simulink model "Integrated_model"  (R2017b)
settings: Solver=VariableStepAuto  StartTime=0.0  StopTime=10.0  RelTol=1e-3
model workspace (MAT data in the model file):
  H_Speed = 3600
  H_limit = 2500
  L_limit = 0
  inputVoltage = 5
  nBitConverter = 10
undefined symbols (not defined in the file): sigbuilder_block
libraries: simulink x2
(part 1 of 2)
settings Model: Creator=ECoDe_user11  LastModifiedBy=ECoDe_user11
settings DebuggingCC: SignalInfNanChecking=warning  ParameterUnderflowMsg=warning  UniqueDataStoreMsg=warning  StrictBusMsg=ErrorOnBusTreatedAsVector

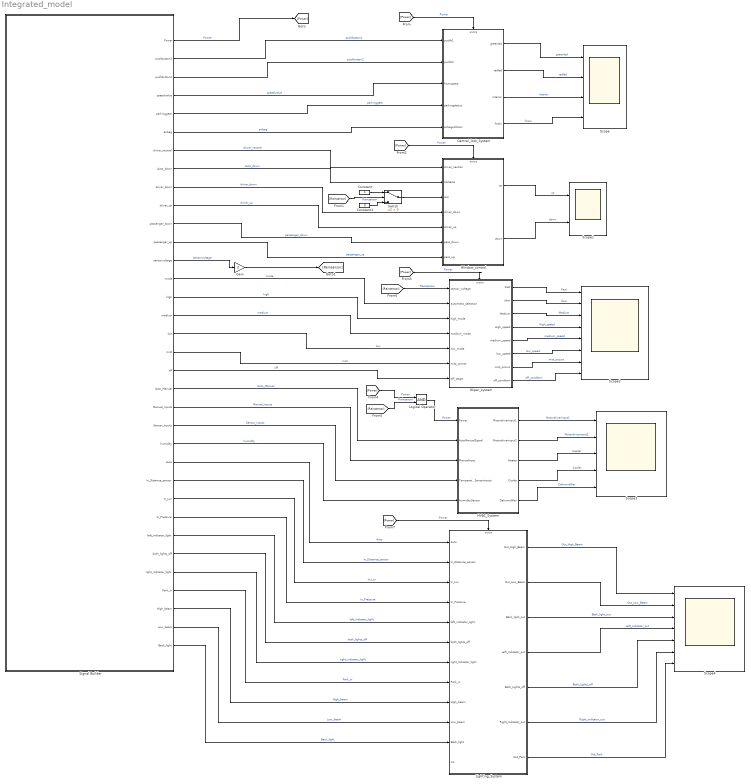
== system Integrated_model ==
  Central_lock_System : Subsystem
  Constant : Constant
  Constant1 : Constant  Value=0
  Gain : Gain  Gain=2
  HVAC_System : Subsystem
  Lighting_System : Subsystem
  Logical Operator : Logic  AllPortsSameDT=off  OutDataTypeStr=boolean
  Scope : Scope  NumInputPorts=4
  Scope1 : Scope  NumInputPorts=2
  Scope2 : Scope  NumInputPorts=8
  Scope3 : Scope  NumInputPorts=5
  Scope4 : Scope  NumInputPorts=7
  Signal Builder : Subsystem  Tag=STV Subsys  LoadFcn=sigbuilder_block('load');  StartFcn=sigbuilder_block('start');  StopFcn=sigbuilder_block('stop');  ClipboardFcn=sigbuilder_block('clipboard');  mask(Sigbuilder block){tuvar=[0:10]}
      mask help: Simulink:masks:SigbuilderBlock_MD
      mask init:
      | if ~strcmp(get_param(bdroot(gcbh),'SimulationStatus'),'stopped') tuvar = sigbuilder_block('maskInit'); end
      settings: CopyFcn=sigbuilder_block('copy');  DeleteFcn=sigbuilder_block('delete');  ModelCloseFcn=sigbuilder_block('modelClose');  PreSaveFcn=sigbuilder_block('preSave');  PauseFcn=sigbuilder_block('pause');  ContinueFcn=sigbuilder_block('continue');  NameChangeFcn=sigbuilder_block('namechange');  OpenFcn=sigbuilder_block('open',[437.25 159 550.5 363.75 ]);  CloseFcn=sigbuilder_block('close');
      mask Display: plot(0, 0, 100, 100,[2, 2, 32, 32, 2], [68, 8, 8, 68, 68],[32, 2], [38, 38], [32, 19, 2],[53, 60, 44], [32, 17, 17, 2],[16, 16, 31, 31]);txt = getActiveGroup(gcbh);text(2, 100, txt,'verticalAlignment', 'top');
  Switch : Switch  Criteria=u2 > Threshold
  Window_control : Subsystem
  Wiper_system : Subsystem
  wires:
  Signal Builder/2(pushbutton1) -> Central_lock_System/1(pushb1)  "pushbutton1"
  Signal Builder/3(pushbutton2) -> Central_lock_System/2(pushb2)  "pushbutton2"
  Signal Builder/4(speedvalue) -> Central_lock_System/3(fromspeed)  "speedvalue"
  Signal Builder/5(parkinggear) -> Central_lock_System/4(parkingstatus)  "parkinggear"
  Signal Builder/6(airbag) -> Central_lock_System/5(airbagcollision)  "airbag"
  Signal Builder/7(driver_neutral) -> Window_control/1(driver_neutral)  "driver_neutral"
  Signal Builder/8(Auto_down) -> Window_control/2(obstacle)  "Auto_down"
  Signal Builder/9(driver_down) -> Window_control/4(driver_down)  "driver_down"
  Signal Builder/10(driver_up) -> Window_control/5(driver_up)  "driver_up"
  Signal Builder/11(passenger_down) -> Window_control/6(pass_down)  "passenger_down"
  Signal Builder/12(passenger_up) -> Window_control/7(pass_up)  "passenger_up"
  Signal Builder/1(Power) -> [Power]  "Power"
  Signal Builder/13(sensorvoltage) -> Gain/1  "sensorvoltage"
  [Power] -> Central_lock_System/Enable  "Power"
  [Power] -> Window_control/Enable  "Power"
  [Power] -> Wiper_system/Enable  "Power"
  [Power] -> Logical Operator/1  "Power"
  [Rainsensor] -> Logical Operator/2  "Rainsensor"
  Switch/1 -> Window_control/3(rain)
  [Rainsensor] -> Switch/2  "Rainsensor"
  Constant/1 -> Switch/1
  Constant1/1 -> Switch/3
  Gain/1 -> [Rainsensor]
  Logical Operator/1 -> HVAC_System/1(Power)  "Power"
  [Rainsensor] -> Wiper_system/1(sensor_voltage)  "Rainsensor"
  Signal Builder/14(mode) -> Wiper_system/2(automatic_selection)  "mode"
  Signal Builder/15(high) -> Wiper_system/3(high_mode)  "high"
  Signal Builder/16(medium) -> Wiper_system/4(medium_mode)  "medium"
  Signal Builder/17(low) -> Wiper_system/5(low_mode)  "low"
  Signal Builder/18(mist) -> Wiper_system/6(mist_comes)  "mist"
  Signal Builder/19(off) -> Wiper_system/7(off_stage)  "off"
  Signal Builder/20(Auto_Manual) -> HVAC_System/2(AutoManualSignal)  "Auto_Manual"
  Signal Builder/21(Manual_inputs) -> HVAC_System/3(ManualInpts)  "Manual_inputs"
  Signal Builder/22(Sensor_inputs) -> HVAC_System/4(TemperatureSensorinputs)  "Sensor_inputs"
  Signal Builder/23(humidity) -> HVAC_System/5(HumiditySensor)  "humidity"
  [Power] -> Lighting_System/Enable  "Power"
  Signal Builder/24(Auto) -> Lighting_System/1(Auto)  "Auto"
  Signal Builder/25(In_Distance_sensor) -> Lighting_System/2(In_Distance_sensor)  "In_Distance_sensor"
  Signal Builder/26(In_Lux) -> Lighting_System/3(In_Lux)  "In_Lux"
  Signal Builder/27(In_Pressure) -> Lighting_System/4(In_Pressure)  "In_Pressure"
  Signal Builder/28(left_indicator_light) -> Lighting_System/5(left_indicator_light)  "left_indicator_light"
  Signal Builder/29(both_lights_off) -> Lighting_System/6(both_lights_off)  "both_lights_off"
  Signal Builder/30(right_indicator_light) -> Lighting_System/7(right_indicator_light)  "right_indicator_light"
  Signal Builder/31(Park_in) -> Lighting_System/8(Park_in)  "Park_in"
  Signal Builder/32(High_beam) -> Lighting_System/9(High_beam)  "High_beam"
  Signal Builder/33(Low_beam) -> Lighting_System/10(Low_beam)  "Low_beam"
  Signal Builder/34(Back_light) -> Lighting_System/11(Back_light)  "Back_light"
  Central_lock_System/1(greenled) -> Scope/1  "greenled"
  Central_lock_System/2(redled) -> Scope/2  "redled"
  Central_lock_System/3(interior) -> Scope/3  "interior"
  Central_lock_System/4(finalv) -> Scope/4  "finalv"
  Window_control/1(up) -> Scope1/1  "up"
  Window_control/2(down) -> Scope1/2  "down"
  Wiper_system/1(Fast) -> Scope2/1  "Fast"
  Wiper_system/2(slow) -> Scope2/2  "slow"
  Wiper_system/3(Medium) -> Scope2/3  "Medium"
  Wiper_system/4(High_speed) -> Scope2/4  "High_speed"
  Wiper_system/5(medium_speed) -> Scope2/5  "medium_speed"
  Wiper_system/6(low_speed) -> Scope2/6  "low_speed"
  Wiper_system/7(mist_occurs) -> Scope2/7  "mist_occurs"
  Wiper_system/8(off_condition) -> Scope2/8  "off_condition"
  HVAC_System/1(Motordriverinput1) -> Scope3/1  "Motordriverinput1"
  HVAC_System/2(Motordriverinput2) -> Scope3/2  "Motordriverinput2"
  HVAC_System/3(Heater) -> Scope3/3  "Heater"
  HVAC_System/4(Cooler) -> Scope3/4  "Cooler"
  HVAC_System/5(Dehumidifier) -> Scope3/5  "Dehumidifier"
  Lighting_System/1(Out_High_Beam) -> Scope4/1  "Out_High_Beam"
  Lighting_System/2(Out_Low_Beam) -> Scope4/2  "Out_Low_Beam"
  Lighting_System/3(Back_light_out) -> Scope4/3  "Back_light_out"
  Lighting_System/4(Left_indicator_out) -> Scope4/4  "Left_indicator_out"
  Lighting_System/5(Both_Lights_off) -> Scope4/5  "Both_Lights_off"
  Lighting_System/6(Right_indicator_out) -> Scope4/6  "Right_indicator_out"
  Lighting_System/7(Out_Park) -> Scope4/7  "Out_Park"

== system Integrated_model/Central_lock_System ==
  note: %REQUIRMENTS:
      | CENTRAL LOCKING SYSTEM
      | CONSISTS OF FOUR SUB SYSTEMS
      | SUB SYSTEM FOR LIGHTING
      | SUB SYSTEM FOR MANUAL
      | SUB SYSTEM FOR AUTOMATIC
      | SUB SYSTEM FOR EMERGENCY
      | INPUTS:
      | PUSHBUTTON1
      | PUSHBUTTON2
      | INPUTBASEDONSPEED
      | INPUTBASEDONPARKINGGEAR
      | AIRBAGINPUT
      | OUTPUTS:
      | LEDS AND INTERIORLIGHTS
      | LOCK AND UNLOCK STATUS
  pushb1 : Inport
  pushb2 : Inport  Port=2
  fromspeed : Inport  Port=3
  parkingstatus : Inport  Port=4
  airbagcollision : Inport  Port=5
  power : EnablePort
  main_locking_system : Subsystem
  greenled : Outport
  redled : Outport  Port=2
  interior : Outport  Port=3
  finalv : Outport  Port=4
  wires:
  fromspeed/1 -> main_locking_system/3(fromspeed)  "fromspeed"
  main_locking_system/2(redled) -> redled/1  "redled"
  main_locking_system/3(interior) -> interior/1  "interior"
  main_locking_system/4(finalv) -> finalv/1  "finalv"
  airbagcollision/1 -> main_locking_system/5(airbagcollision)  "airbagcollision"
  parkingstatus/1 -> main_locking_system/4(parkingstatus)  "parkingstatus"
  main_locking_system/1(greenled) -> greenled/1  "greenled"
  pushb2/1 -> main_locking_system/2(pushb2)  "pushb2"
  pushb1/1 -> main_locking_system/1(pushb1)  "pushb1"

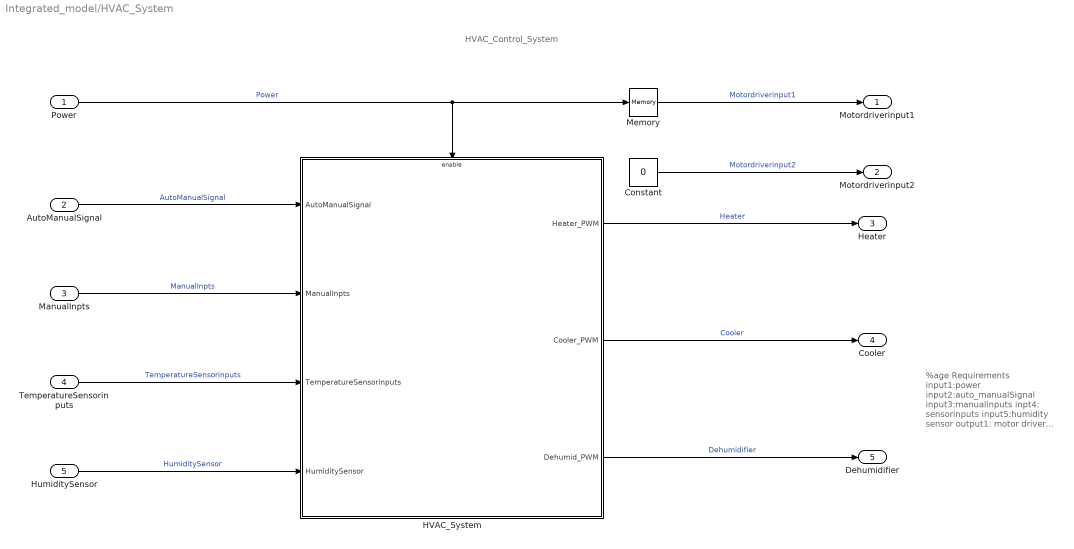
== system Integrated_model/HVAC_System ==
  note: HVAC_Control_System
  note: %age Requirements
      |
      | input1:power
      | input2:auto_manualSignal
      | input3:manualinputs
      | inpt4: sensorinputs
      | input5:humidity sensor
      | output1: motor driver output
      | output2: mptor driver output
      | output3: PWM for Heater
      | output4: PWM for Cooler
      | output5: PWM for Dehumidifier
  Power : Inport
  AutoManualSignal : Inport  Port=2
  ManualInpts : Inport  Port=3
  TemperatureSensorinputs : Inport  Port=4
  HumiditySensor : Inport  Port=5
  Constant : Constant  Value=0
  HVAC_System : Subsystem
  Memory : Memory
  Motordriverinput1 : Outport
  Motordriverinput2 : Outport  Port=2
  Heater : Outport  Port=3
  Cooler : Outport  Port=4
  Dehumidifier : Outport  Port=5
  wires:
  AutoManualSignal/1 -> HVAC_System/1(AutoManualSignal)  "AutoManualSignal"
  ManualInpts/1 -> HVAC_System/2(ManualInpts)  "ManualInpts"
  TemperatureSensorinputs/1 -> HVAC_System/3(TemperatureSensorinputs)  "TemperatureSensorinputs"
  Power/1 -> Memory/1, HVAC_System/Enable  "Power"
  HVAC_System/1(Heater_PWM) -> Heater/1  "Heater"
  HVAC_System/3(Dehumid_PWM) -> Dehumidifier/1  "Dehumidifier"
  HumiditySensor/1 -> HVAC_System/4(HumiditySensor)  "HumiditySensor"
  HVAC_System/2(Cooler_PWM) -> Cooler/1  "Cooler"
  Constant/1 -> Motordriverinput2/1  "Motordriverinput2"
  Memory/1 -> Motordriverinput1/1  "Motordriverinput1"

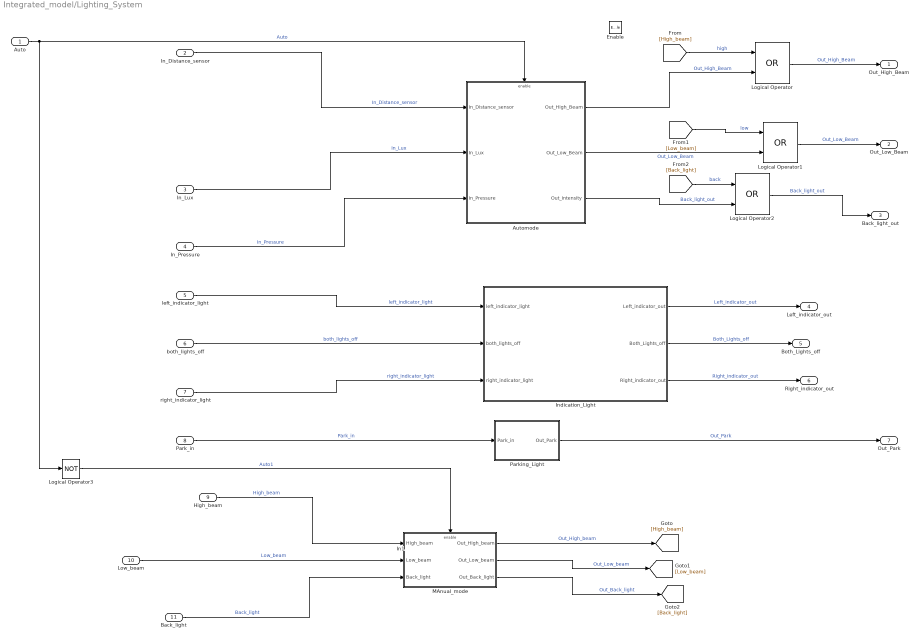
== system Integrated_model/Lighting_System ==
  Auto : Inport
  In_Distance_sensor : Inport  Port=2
  In_Lux : Inport  Port=3
  In_Pressure : Inport  Port=4
  left_indicator_light : Inport  Port=5
  both_lights_off : Inport  Port=6
  right_indicator_light : Inport  Port=7
  Park_in : Inport  Port=8
  High_beam : Inport  Port=9
  Low_beam : Inport  Port=10
  Back_light : Inport  Port=11
  In1 : Inport  Port=12
  Enable : EnablePort
  Automode : Subsystem
  Indication_Light : Subsystem
  Logical Operator : Logic  Operator=OR  AllPortsSameDT=off  OutDataTypeStr=boolean
  Logical Operator1 : Logic  Operator=OR  AllPortsSameDT=off  OutDataTypeStr=boolean
  Logical Operator2 : Logic  Operator=OR  AllPortsSameDT=off  OutDataTypeStr=boolean
  Logical Operator3 : Logic  Operator=NOT  AllPortsSameDT=off  OutDataTypeStr=boolean
  MAnual_mode : Subsystem
  Parking_Light : Subsystem
  Out_High_Beam : Outport
  Out_Low_Beam : Outport  Port=2
  Back_light_out : Outport  Port=3
  Left_indicator_out : Outport  Port=4
  Both_Lights_off : Outport  Port=5
  Right_indicator_out : Outport  Port=6
  Out_Park : Outport  Port=7
  wires:
  both_lights_off/1 -> Indication_Light/2(both_lights_off)  "both_lights_off"
  left_indicator_light/1 -> Indication_Light/1(left_indicator_light)  "left_indicator_light"
  Park_in/1 -> Parking_Light/1(Park_in)  "Park_in"
  Parking_Light/1(Out_Park) -> Out_Park/1  "Out_Park"
  right_indicator_light/1 -> Indication_Light/3(right_indicator_light)  "right_indicator_light"
  Indication_Light/1(Left_indicator_out) -> Left_indicator_out/1  "Left_indicator_out"
  Indication_Light/2(Both_Lights_off) -> Both_Lights_off/1  "Both_Lights_off"
  Indication_Light/3(Right_indicator_out) -> Right_indicator_out/1  "Right_indicator_out"
  In_Distance_sensor/1 -> Automode/1(In_Distance_sensor)  "In_Distance_sensor"
  In_Lux/1 -> Automode/2(In_Lux)  "In_Lux"
  In_Pressure/1 -> Automode/3(In_Pressure)  "In_Pressure"
  Auto/1 -> Automode/Enable, Logical Operator3/1  "Auto"
  [High_beam] -> Logical Operator/1  "high"
  Automode/1(Out_High_Beam) -> Logical Operator/2  "Out_High_Beam"
  Logical Operator/1 -> Out_High_Beam/1  "Out_High_Beam"
  Automode/2(Out_Low_Beam) -> Logical Operator1/2  "Out_Low_Beam"
  [Low_beam] -> Logical Operator1/1  "low"
  Logical Operator1/1 -> Out_Low_Beam/1  "Out_Low_Beam"
  [Back_light] -> Logical Operator2/1  "back"
  Automode/3(Out_Intensity) -> Logical Operator2/2  "Back_light_out"
  Logical Operator2/1 -> Back_light_out/1  "Back_light_out"
  High_beam/1 -> MAnual_mode/1(High_beam)  "High_beam"
  Low_beam/1 -> MAnual_mode/2(Low_beam)  "Low_beam"
  Back_light/1 -> MAnual_mode/3(Back_light)  "Back_light"
  MAnual_mode/1(Out_High_beam) -> [High_beam]  "Out_High_beam"
  MAnual_mode/2(Out_Low_beam) -> [Low_beam]  "Out_Low_beam"
  MAnual_mode/3(Out_Back_light) -> [Back_light]  "Out_Back_light"
  Logical Operator3/1 -> MAnual_mode/Enable  "Auto1"

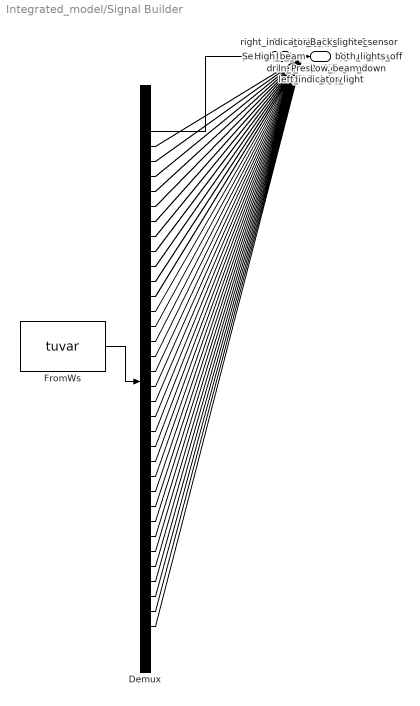
== system Integrated_model/Signal Builder ==
  Demux : Demux  Tag=STV Demux  Outputs=34
  FromWs : FromWorkspace  Tag=STV FromWs  VariableName=tuvar  SampleTime=0
      SigBuilderData=|
      | common.afterFinalStr = 'Extrapolate'
      | common.sampleTime = 0
      | dataSet.timeRange = [0 0.1]
      | dataSet.name = 'Sheet1'
      | sbobj.Name = 'Signal Builder'
      | sbobj.Groups.Name = 'Sheet1'
      | sbobj.Groups.Signals(1).Name = 'Power'
      | sbobj.Groups.Signals(1).XData = [0 0.1]
      | sbobj.Groups.Signals(1).YData = [0 0]
      | sbobj.Groups.Signals(2).Name = 'pushbutton1'
      | sbobj.Groups.Signals(2).XData = [0 0.1]
      | sbobj.Groups.Signals(2).YData = [0 0]
      | sbobj.Groups.Signals(3).Name = 'pushbutton2'
      | sbobj.Groups.Signals(3).XData = [0 0.1]
      | sbobj.Groups.Signals(3).YData = [0 0]
      | sbobj.Groups.Signals(4).Name = 'speedvalue'
      | sbobj.Groups.Signals(4).XData = [0 0.1]
      | sbobj.Groups.Signals(4).YData = [0 0]
      | sbobj.Groups.Signals(5).Name = 'parkinggear'
      | sbobj.Groups.Signals(5).XData = [0 0.1]
      | sbobj.Groups.Signals(5).YData = [0 0]
      | sbobj.Groups.Signals(6).Name = 'airbag'
      | sbobj.Groups.Signals(6).XData = [0 0.1]
      | sbobj.Groups.Signals(6).YData = [0 0]
      | sbobj.Groups.Signals(7).Name = 'driver_neutral'
      | sbobj.Groups.Signals(7).XData = [0 0.1]
      | sbobj.Groups.Signals(7).YData = [0 0]
      | sbobj.Groups.Signals(8).Name = 'Auto_down'
      | sbobj.Groups.Signals(8).XData = [0 0.1]
      | sbobj.Groups.Signals(8).YData = [0 0]
      | sbobj.Groups.Signals(9).Name = 'driver_down'
      | sbobj.Groups.Signals(9).XData = [0 0.1]
      | sbobj.Groups.Signals(9).YData = [0 0]
      | sbobj.Groups.Signals(10).Name = 'driver_up'
      | sbobj.Groups.Signals(10).XData = [0 0.1]
      | sbobj.Groups.Signals(10).YData = [0 0]
      | sbobj.Groups.Signals(11).Name = 'passenger_down'
      | sbobj.Groups.Signals(11).XData = [0 0.1]
      | sbobj.Groups.Signals(11).YData = [0 0]
      | sbobj.Groups.Signals(12).Name = 'passenger_up'
      | sbobj.Groups.Signals(12).XData = [0 0.1]
      | sbobj.Groups.Signals(12).YData = [0 0]
      | sbobj.Groups.Signals(13).Name = 'sensorvoltage'
      | sbobj.Groups.Signals(13).XData = [0 0.1]
      | sbobj.Groups.Signals(13).YData = [0 0]
      | sbobj.Groups.Signals(14).Name = 'mode'
      | sbobj.Groups.Signals(14).XData = [0 0.1]
      | sbobj.Groups.Signals(14).YData = [0 0]
      | sbobj.Groups.Signals(15).Name = 'high'
      | sbobj.Groups.Signals(15).XData = [0 0.1]
      | sbobj.Groups.Signals(15).YData = [0 0]
      | sbobj.Groups.Signals(16).Name = 'medium'
      | sbobj.Groups.Signals(16).XData = [0 0.1]
      | sbobj.Groups.Signals(16).YData = [0 0]
      | sbobj.Groups.Signals(17).Name = 'low'
      | sbobj.Groups.Signals(17).XData = [0 0.1]
      | sbobj.Groups.Signals(17).YData = [0 0]
      | sbobj.Groups.Signals(18).Name = 'mist'
      | sbobj.Groups.Signals(18).XData = [0 0.1]
      | sbobj.Groups.Signals(18).YData = [0 0]
      | sbobj.Groups.Signals(19).Name = 'off'
      | sbobj.Groups.Signals(19).XData = [0 0.1]
      | sbobj.Groups.Signals(19).YData = [0 0]
      | sbobj.Groups.Signals(20).Name = 'Auto_Manual'
      | sbobj.Groups.Signals(20).XData = [0 0.1]
      | sbobj.Groups.Signals(20).YData = [0 0]
      | sbobj.Groups.Signals(21).Name = 'Manual_inputs'
      | sbobj.Groups.Signals(21).XData = [0 0.1]
      | sbobj.Groups.Signals(21).YData = [0 0]
      | sbobj.Groups.Signals(22).Name = 'Sensor_inputs'
      | sbobj.Groups.Signals(22).XData = [0 0.1]
      | sbobj.Groups.Signals(22).YData = [0 0]
      | sbobj.Groups.Signals(23).Name = 'humidity'
      | sbobj.Groups.Signals(23).XData = [0 0.1]
      | sbobj.Groups.Signals(23).YData = [0 0]
      | sbobj.Groups.Signals(24).Name = 'Auto'
      | sbobj.Groups.Signals(24).XData = [0 0.1]
      | sbobj.Groups.Signals(24).YData = [0 0]
      | sbobj.Groups.Signals(25).Name = 'In_Distance_sensor'
      | sbobj.Groups.Signals(25).XData = [0 0.1]
      | sbobj.Groups.Signals(25).YData = [0 0]
      | sbobj.Groups.Signals(26).Name = 'In_Lux'
      | sbobj.Groups.Signals(26).XData = [0 0.1]
      | sbobj.Groups.Signals(26).YData = [0 0]
      | sbobj.Groups.Signals(27).Name = 'In_Pressure'
      | sbobj.Groups.Signals(27).XData = [0 0.1]
      | sbobj.Groups.Signals(27).YData = [0 0]
      | sbobj.Groups.Signals(28).Name = 'left_indicator_light'
      | sbobj.Groups.Signals(28).XData = [0 0.1]
      | sbobj.Groups.Signals(28).YData = [0 0]
      | sbobj.Groups.Signals(29).Name = 'both_lights_off'
      | sbobj.Groups.Signals(29).XData = [0 0.1]
      | sbobj.Groups.Signals(29).YData = [0 0]
      | sbobj.Groups.Signals(30).Name = 'right_indicator_light'
      | sbobj.Groups.Signals(30).XData = [0 0.1]
      | sbobj.Groups.Signals(30).YData = [0 0]
      | sbobj.Groups.Signals(31).Name = 'Park_in'
      | sbobj.Groups.Signals(31).XData = [0 0.1]
      | sbobj.Groups.Signals(31).YData = [0 0]
      | sbobj.Groups.Signals(32).Name = 'High_beam'
      | sbobj.Groups.Signals(32).XData = [0 0.1]
      | sbobj.Groups.Signals(32).YData = [0 0]
      | sbobj.Groups.Signals(33).Name = 'Low_beam'
      | sbobj.Groups.Signals(33).XData = [0 0.1]
      | sbobj.Groups.Signals(33).YData = [0 0]
      | sbobj.Groups.Signals(34).Name = 'Back_light'
      | sbobj.Groups.Signals(34).XData = [0 0.1]
      | sbobj.Groups.Signals(34).YData = [0 0]
      | sbobj.Groups.TimeRange = [0 0.1]
  Power : Outport  Tag=STV Outport
  pushbutton1 : Outport  Tag=STV Outport  Port=2
  pushbutton2 : Outport  Tag=STV Outport  Port=3
  speedvalue : Outport  Tag=STV Outport  Port=4
  parkinggear : Outport  Tag=STV Outport  Port=5
  airbag : Outport  Tag=STV Outport  Port=6
  driver_neutral : Outport  Tag=STV Outport  Port=7
  Auto_down : Outport  Tag=STV Outport  Port=8
  driver_down : Outport  Tag=STV Outport  Port=9
  driver_up : Outport  Tag=STV Outport  Port=10
  passenger_down : Outport  Tag=STV Outport  Port=11
  passenger_up : Outport  Tag=STV Outport  Port=12
  sensorvoltage : Outport  Tag=STV Outport  Port=13
  mode : Outport  Tag=STV Outport  Port=14
  high : Outport  Tag=STV Outport  Port=15
  medium : Outport  Tag=STV Outport  Port=16
  low : Outport  Tag=STV Outport  Port=17
  mist : Outport  Tag=STV Outport  Port=18
  off : Outport  Tag=STV Outport  Port=19
  Auto_Manual : Outport  Tag=STV Outport  Port=20
  Manual_inputs : Outport  Tag=STV Outport  Port=21
  Sensor_inputs : Outport  Tag=STV Outport  Port=22
  humidity : Outport  Tag=STV Outport  Port=23
  Auto : Outport  Tag=STV Outport  Port=24
  In_Distance_sensor : Outport  Tag=STV Outport  Port=25
  In_Lux : Outport  Tag=STV Outport  Port=26
  In_Pressure : Outport  Tag=STV Outport  Port=27
  left_indicator_light : Outport  Tag=STV Outport  Port=28
  both_lights_off : Outport  Tag=STV Outport  Port=29
  right_indicator_light : Outport  Tag=STV Outport  Port=30
  Park_in : Outport  Tag=STV Outport  Port=31
  High_beam : Outport  Tag=STV Outport  Port=32
  Low_beam : Outport  Tag=STV Outport  Port=33
  Back_light : Outport  Tag=STV Outport  Port=34
  wires:
  Demux/1 -> Power/1
  FromWs/1 -> Demux/1
  Demux/2 -> pushbutton1/1
  Demux/3 -> pushbutton2/1
  Demux/4 -> speedvalue/1
  Demux/5 -> parkinggear/1
  Demux/6 -> airbag/1
  Demux/7 -> driver_neutral/1
  Demux/8 -> Auto_down/1
  Demux/9 -> driver_down/1
  Demux/10 -> driver_up/1
  Demux/11 -> passenger_down/1
  Demux/12 -> passenger_up/1
  Demux/13 -> sensorvoltage/1
  Demux/14 -> mode/1
  Demux/15 -> high/1
  Demux/16 -> medium/1
  Demux/17 -> low/1
  Demux/18 -> mist/1
  Demux/19 -> off/1
  Demux/20 -> Auto_Manual/1
  Demux/21 -> Manual_inputs/1
  Demux/22 -> Sensor_inputs/1
  Demux/23 -> humidity/1
  Demux/24 -> Auto/1
  Demux/25 -> In_Distance_sensor/1
  Demux/26 -> In_Lux/1
  Demux/27 -> In_Pressure/1
  Demux/28 -> left_indicator_light/1
  Demux/29 -> both_lights_off/1
  Demux/30 -> right_indicator_light/1
  Demux/31 -> Park_in/1
  Demux/32 -> High_beam/1
  Demux/33 -> Low_beam/1
  Demux/34 -> Back_light/1

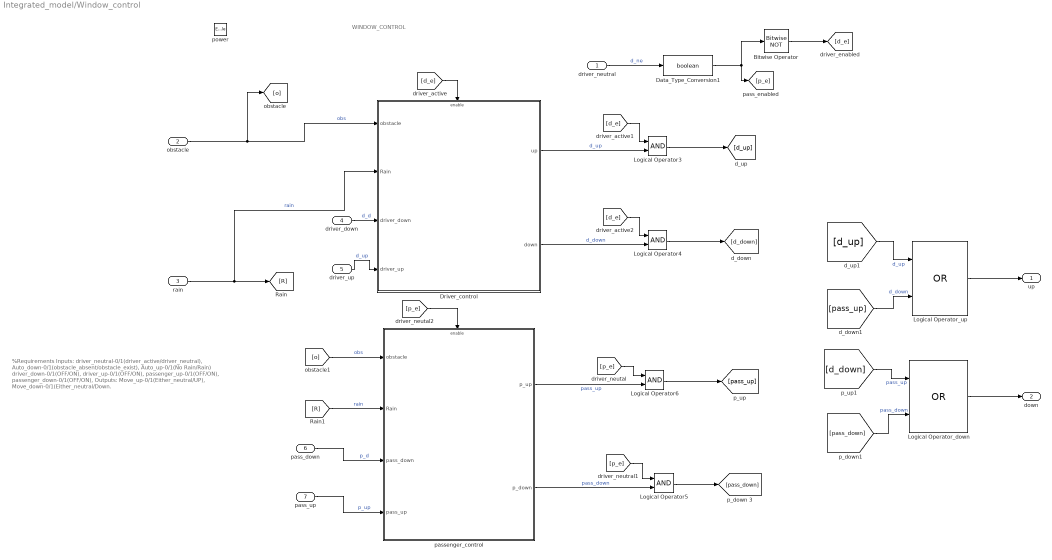
== system Integrated_model/Window_control ==
  note: %Requirements
      | Inputs:
      | driver_neutral-0/1(driver_active/driver_neutral),
      | Auto_down-0/1(obstacle_absent/obstacle_exist),
      | Auto_up-0/1(No Rain/Rain)
      | driver_down-0/1(OFF/ON),
      | driver_up-0/1(OFF/ON),
      | passenger_up-0/1(OFF/ON),
      | passenger_down-0/1(OFF/ON),
      | Outputs:
      | Move_up-0/1(Either_neutral/UP),
      | Move_down-0/1(Either_neutral/Down.
  note: WINDOW_CONTROL
  driver_neutral : Inport
  obstacle : Inport  Port=2
  rain : Inport  Port=3
  driver_down : Inport  Port=4
  driver_up : Inport  Port=5
  pass_down : Inport  Port=6
  pass_up : Inport  Port=7
  power : EnablePort
  Bitwise Operator : simulink/Logic and Bit Operations/Bitwise Operator  logicop=NOT  UseBitMask=off  BitMask=bin2dec('11011001')  BitMaskRealWorld=Stored Integer
  Data_Type_Conversion1 : DataTypeConversion  OutDataTypeStr=boolean
  Driver_control : Subsystem
  Logical Operator{3..6} (4 alike) : Logic  AllPortsSameDT=off  OutDataTypeStr=boolean
  Logical Operator_down : Logic  Operator=OR  AllPortsSameDT=off  OutDataTypeStr=boolean
  "Logical Operator_up " : Logic  Operator=OR  AllPortsSameDT=off  OutDataTypeStr=boolean
  passenger_control : Subsystem
  up : Outport
  down : Outport  Port=2
  wires:
  Logical Operator_down/1 -> down/1
  "Logical Operator_up "/1 -> up/1
  Driver_control/1(up) -> Logical Operator3/2  "d_up"
  driver_up/1 -> Driver_control/4(driver_up)  "d_up"
  driver_down/1 -> Driver_control/3(driver_down)  "d_d"
  rain/1 -> [R], Driver_control/2(Rain)  "rain"
  obstacle/1 -> [o], Driver_control/1(obstacle)  "obs"
  pass_down/1 -> passenger_control/3(pass_down)  "p_d"
  pass_up/1 -> passenger_control/4(pass_up)  "p_up"
  Driver_control/2(down) -> Logical Operator4/2  "d_down"
  driver_neutral/1 -> Data_Type_Conversion1/1  "d_ne"
  Data_Type_Conversion1/1 -> [p_e], Bitwise Operator/1
  passenger_control/1(p_up) -> Logical Operator6/2  "pass_up"
  passenger_control/2(p_down) -> Logical Operator5/2  "pass_down"
  [p_e] -> passenger_control/Enable
  [p_e] -> Logical Operator6/1
  [p_e] -> Logical Operator5/1
  Bitwise Operator/1 -> [d_e]
  [d_e] -> Driver_control/Enable
  [d_e] -> Logical Operator3/1
  [d_e] -> Logical Operator4/1
  Logical Operator3/1 -> [d_up]
  Logical Operator6/1 -> [pass_up]
  Logical Operator5/1 -> [pass_down]
  Logical Operator4/1 -> [d_down]
  [d_up] -> "Logical Operator_up "/1  "d_up"
  [pass_up] -> "Logical Operator_up "/2  "d_down"
  [d_down] -> Logical Operator_down/1  "pass_up"
  [pass_down] -> Logical Operator_down/2  "pass_down"
  [o] -> passenger_control/1(obstacle)  "obs"
  [R] -> passenger_control/2(Rain)  "rain"

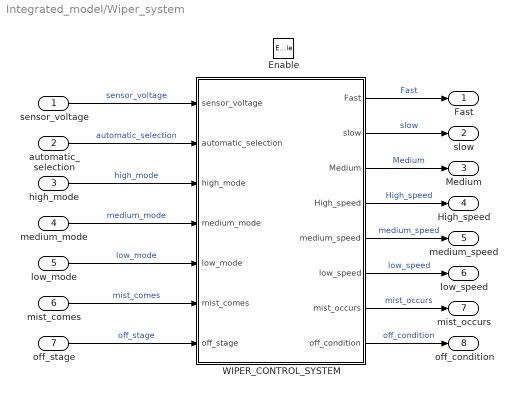
== system Integrated_model/Wiper_system ==
  sensor_voltage : Inport
  automatic_selection : Inport  Port=2
  high_mode : Inport  Port=3
  medium_mode : Inport  Port=4
  low_mode : Inport  Port=5
  mist_comes : Inport  Port=6
  off_stage : Inport  Port=7
  Enable : EnablePort
  WIPER_CONTROL_SYSTEM : Subsystem
  Fast : Outport
  slow : Outport  Port=2
  Medium : Outport  Port=3
  High_speed : Outport  Port=4
  medium_speed : Outport  Port=5
  low_speed : Outport  Port=6
  mist_occurs : Outport  Port=7
  off_condition : Outport  Port=8
  wires:
  off_stage/1 -> WIPER_CONTROL_SYSTEM/7(off_stage)  "off_stage"
  WIPER_CONTROL_SYSTEM/5(medium_speed) -> medium_speed/1  "medium_speed"
  WIPER_CONTROL_SYSTEM/1(Fast) -> Fast/1  "Fast"
  WIPER_CONTROL_SYSTEM/4(High_speed) -> High_speed/1  "High_speed"
  WIPER_CONTROL_SYSTEM/2(slow) -> slow/1  "slow"
  low_mode/1 -> WIPER_CONTROL_SYSTEM/5(low_mode)  "low_mode"
  high_mode/1 -> WIPER_CONTROL_SYSTEM/3(high_mode)  "high_mode"
  WIPER_CONTROL_SYSTEM/7(mist_occurs) -> mist_occurs/1  "mist_occurs"
  automatic_selection/1 -> WIPER_CONTROL_SYSTEM/2(automatic_selection)  "automatic_selection"
  WIPER_CONTROL_SYSTEM/6(low_speed) -> low_speed/1  "low_speed"
  medium_mode/1 -> WIPER_CONTROL_SYSTEM/4(medium_mode)  "medium_mode"
  sensor_voltage/1 -> WIPER_CONTROL_SYSTEM/1(sensor_voltage)  "sensor_voltage"
  mist_comes/1 -> WIPER_CONTROL_SYSTEM/6(mist_comes)  "mist_comes"
  WIPER_CONTROL_SYSTEM/8(off_condition) -> off_condition/1  "off_condition"
  WIPER_CONTROL_SYSTEM/3(Medium) -> Medium/1  "Medium"

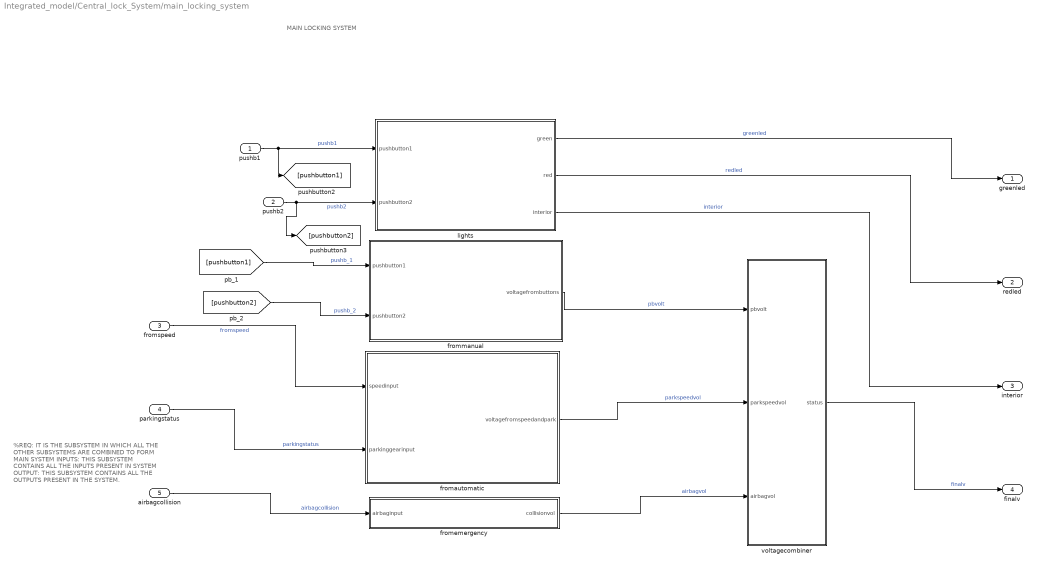
== system Integrated_model/Central_lock_System/main_locking_system ==
  note: %REQ:
      | IT IS THE SUBSYSTEM IN
      | WHICH ALL THE OTHER SUBSYSTEMS
      | ARE COMBINED TO FORM MAIN SYSTEM
      | INPUTS:
      | THIS SUBSYSTEM CONTAINS ALL THE
      | INPUTS PRESENT IN SYSTEM
      | OUTPUT:
      | THIS SUBSYSTEM CONTAINS ALL THE
      | OUTPUTS PRESENT IN  THE SYSTEM.
  note: MAIN LOCKING SYSTEM
  pushb1 : Inport
  pushb2 : Inport  Port=2
  fromspeed : Inport  Port=3
  parkingstatus : Inport  Port=4
  airbagcollision : Inport  Port=5
  fromautomatic : Subsystem
  fromemergency : Subsystem
  frommanual : Subsystem
  lights : Subsystem
  voltagecombiner : Subsystem
  greenled : Outport
  redled : Outport  Port=2
  interior : Outport  Port=3
  finalv : Outport  Port=4
  wires:
  pushb1/1 -> [pushbutton1], lights/1(pushbutton1)  "pushb1"
  voltagecombiner/1(status) -> finalv/1  "finalv"
  frommanual/1(voltagefrombuttons) -> voltagecombiner/1(pbvolt)  "pbvolt"
  airbagcollision/1 -> fromemergency/1(airbaginput)  "airbagcollision"
  fromautomatic/1(voltagefromspeedandpark) -> voltagecombiner/2(parkspeedvol)  "parkspeedvol"
  [pushbutton1] -> frommanual/1(pushbutton1)  "pushb_1"
  pushb2/1 -> [pushbutton2], lights/2(pushbutton2)  "pushb2"
  parkingstatus/1 -> fromautomatic/2(parkinggearinput)  "parkingstatus"
  fromspeed/1 -> fromautomatic/1(speedinput)  "fromspeed"
  lights/1(green) -> greenled/1  "greenled"
  lights/3(interior) -> interior/1  "interior"
  lights/2(red) -> redled/1  "redled"
  fromemergency/1(collisionvol) -> voltagecombiner/3(airbagvol)  "airbagvol"
  [pushbutton2] -> frommanual/2(pushbutton2)  "pushb_2"

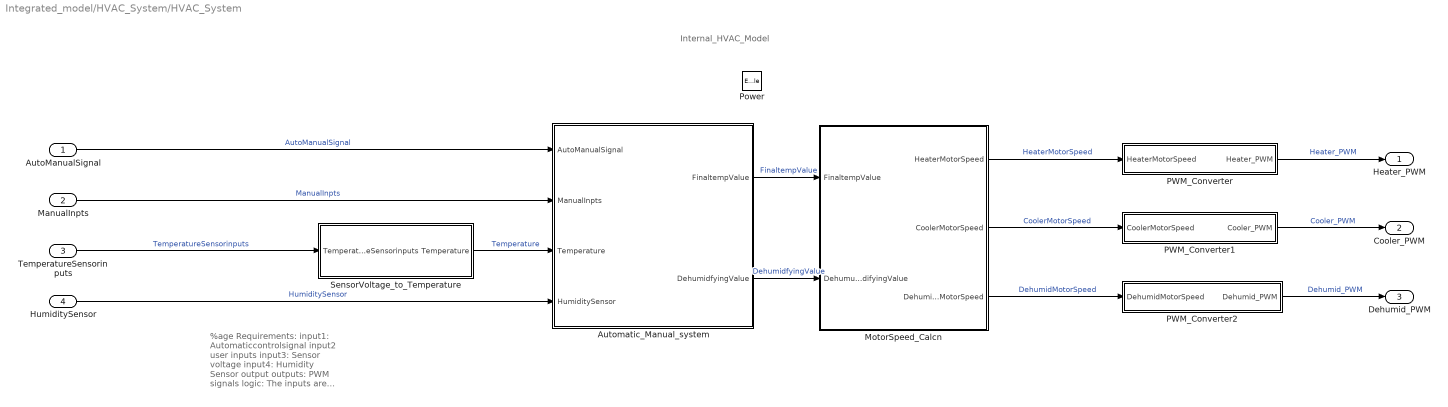
== system Integrated_model/HVAC_System/HVAC_System ==
  note: Internal_HVAC_Model
  note: %age Requirements:
      |
      | input1: Automaticcontrolsignal
      | input2 user inputs
      | input3: Sensor voltage
      | input4: Humidity Sensor output
      | outputs: PWM signals
      | logic: The inputs are converted to the required
      | motor PWMs which will given to respective motors
  AutoManualSignal : Inport
  ManualInpts : Inport  Port=2
  TemperatureSensorinputs : Inport  Port=3
  HumiditySensor : Inport  Port=4
  Power : EnablePort
  Automatic_Manual_system : Subsystem
  MotorSpeed_Calcn : Subsystem
  PWM_Converter : Subsystem
  PWM_Converter1 : Subsystem
  PWM_Converter2 : Subsystem
  SensorVoltage_to_Temperature : Subsystem
  Heater_PWM : Outport
  Cooler_PWM : Outport  Port=2
  Dehumid_PWM : Outport  Port=3
  wires:
  Automatic_Manual_system/2(DehumidfyingValue) -> MotorSpeed_Calcn/2(DehumudifyingValue)  "DehumidfyingValue"
  Automatic_Manual_system/1(FinaltempValue) -> MotorSpeed_Calcn/1(FinaltempValue)  "FinaltempValue"
  PWM_Converter1/1(Cooler_PWM) -> Cooler_PWM/1  "Cooler_PWM"
  TemperatureSensorinputs/1 -> SensorVoltage_to_Temperature/1(TemperatureSensorinputs)  "TemperatureSensorinputs"
  ManualInpts/1 -> Automatic_Manual_system/2(ManualInpts)  "ManualInpts"
  PWM_Converter/1(Heater_PWM) -> Heater_PWM/1  "Heater_PWM"
  SensorVoltage_to_Temperature/1(Temperature) -> Automatic_Manual_system/3(Temperature)  "Temperature"
  PWM_Converter2/1(Dehumid_PWM) -> Dehumid_PWM/1  "Dehumid_PWM"
  MotorSpeed_Calcn/2(CoolerMotorSpeed) -> PWM_Converter1/1(CoolerMotorSpeed)  "CoolerMotorSpeed"
  MotorSpeed_Calcn/1(HeaterMotorSpeed) -> PWM_Converter/1(HeaterMotorSpeed)  "HeaterMotorSpeed"
  AutoManualSignal/1 -> Automatic_Manual_system/1(AutoManualSignal)  "AutoManualSignal"
  MotorSpeed_Calcn/3(DehumidMotorSpeed) -> PWM_Converter2/1(DehumidMotorSpeed)  "DehumidMotorSpeed"
  HumiditySensor/1 -> Automatic_Manual_system/4(HumiditySensor)  "HumiditySensor"

== system Integrated_model/Lighting_System/Automode ==
  In_Distance_sensor : Inport
  In_Lux : Inport  Port=2
  In_Pressure : Inport  Port=3
  Auto : EnablePort
  Conversion_system : Subsystem
  For_BackLight : Subsystem
  HeadLight_and_DayLight : Subsystem
  Light_Indicator_ : Subsystem
  Out_High_Beam : Outport
  Out_Low_Beam : Outport  Port=2
  Out_Intensity : Outport  Port=3
  wires:
  For_BackLight/1(Out_Intensity) -> Out_Intensity/1  "Out_Intensity"
  In_Lux/1 -> Conversion_system/1(In_Lux), Light_Indicator_/1(In_Lux)  "In_Lux"
  HeadLight_and_DayLight/2(Out_Low_Beam) -> Out_Low_Beam/1  "Out_Low_Beam"
  In_Pressure/1 -> For_BackLight/1(In_Pressure)  "In_Pressure"
  In_Distance_sensor/1 -> HeadLight_and_DayLight/1(In_Distance_sensor)  "In_Distance_sensor"
  HeadLight_and_DayLight/1(Out_High_Beam) -> Out_High_Beam/1  "Out_High_Beam"
  Light_Indicator_/1(In_Light_Intensity) -> HeadLight_and_DayLight/4(In_Light_Intensity)  "In_Light_Intensity"
  Conversion_system/2(In_Reflection_opposite_vehicle) -> HeadLight_and_DayLight/3(In_Reflection_opposite_vehicle)  "In_Reflection_opposite_vehicle"
  Conversion_system/1(In_Street_Light) -> HeadLight_and_DayLight/2(In_Street_Light)  "In_Street_Light"

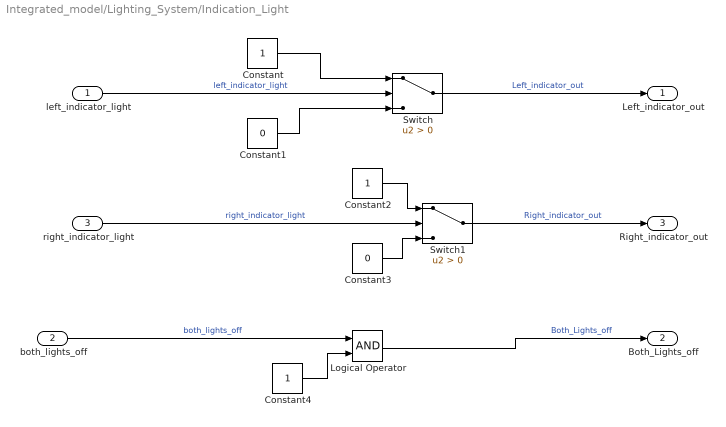
== system Integrated_model/Lighting_System/Indication_Light ==
  left_indicator_light : Inport
  both_lights_off : Inport  Port=2
  right_indicator_light : Inport  Port=3
  Constant : Constant
  Constant1 : Constant  Value=0
  Constant2 : Constant
  Constant3 : Constant  Value=0
  Constant4 : Constant
  Logical Operator : Logic  AllPortsSameDT=off  OutDataTypeStr=boolean
  Switch : Switch  Criteria=u2 > Threshold
  Switch1 : Switch  Criteria=u2 > Threshold
  Left_indicator_out : Outport
  Both_Lights_off : Outport  Port=2
  Right_indicator_out : Outport  Port=3
  wires:
  left_indicator_light/1 -> Switch/2  "left_indicator_light"
  Constant/1 -> Switch/1
  Constant1/1 -> Switch/3
  Constant3/1 -> Switch1/3
  right_indicator_light/1 -> Switch1/2  "right_indicator_light"
  Constant2/1 -> Switch1/1
  Switch/1 -> Left_indicator_out/1  "Left_indicator_out"
  Switch1/1 -> Right_indicator_out/1  "Right_indicator_out"
  Constant4/1 -> Logical Operator/2
  both_lights_off/1 -> Logical Operator/1  "both_lights_off"
  Logical Operator/1 -> Both_Lights_off/1  "Both_Lights_off"

== system Integrated_model/Lighting_System/MAnual_mode ==
  High_beam : Inport
  Low_beam : Inport  Port=2
  Back_light : Inport  Port=3
  Auto1 : EnablePort
  Out_High_beam : Outport
  Out_Low_beam : Outport  Port=2
  Out_Back_light : Outport  Port=3
  wires:
  High_beam/1 -> Out_High_beam/1  "High_beam"
  Low_beam/1 -> Out_Low_beam/1  "Low_beam"
  Back_light/1 -> Out_Back_light/1  "Back_light"

== system Integrated_model/Lighting_System/Parking_Light ==
  Park_in : Inport
  Compare_with_Light : Switch  Criteria=u2 > Threshold
  Lower_Limit : Constant  Value=0
  Out_Park : Outport
  wires:
  Park_in/1 -> Compare_with_Light/1, Compare_with_Light/2  "Park_in"
  Lower_Limit/1 -> Compare_with_Light/3  "Lower_Limit"
  Compare_with_Light/1 -> Out_Park/1  "Out_Park"

== system Integrated_model/Window_control/Driver_control ==
  note: %Requirements
      | Inputs:
      | Obstacle-0/1(obstacle_absent/obstacle_exist),
      | Rain-0/1(No Rain/Rain)
      | driver_down-0/1(OFF/ON),
      | driver_up-0/1(OFF/ON),
      |
      | Outputs:
      | Driver_up-0/1(Either_neutral/UP),
      | Driver_down-0/1(Either_neutral/Down.
  note: DRIVER_WINDOWS_CONTROL
  obstacle : Inport
  Rain : Inport  Port=2
  driver_down : Inport  Port=3
  driver_up : Inport  Port=4
  driver_active : EnablePort
  driver : Stateflow chart  TreatAsAtomicUnit=on
  up : Outport
  down : Outport  Port=2
  wires:
  driver_up/1 -> driver/4(d_up)  "driver_up"
  driver/1(Up) -> up/1  "up"
  driver/2(Down) -> down/1  "down"
  obstacle/1 -> driver/1(Obstacle)  "obstacle"
  Rain/1 -> driver/2(Rain)  "Rain"
  driver_down/1 -> driver/3(d_down)  "driver_down"

== system Integrated_model/Window_control/passenger_control ==
  note: %Requirements
      | Inputs:
      | Obstacle-0/1(obstacle_absent/obstacle_exist),
      | Rain-0/1(No Rain/Rain)
      | passenger_up-0/1(OFF/ON),
      | passenger_down-0/1(OFF/ON),
      | Outputs:
      | Pass_up-0/1(Either_neutral/UP),
      | Pass_down-0/1(Either_neutral/Down.
  note: PASSENGER_WINDOWS_CONTROL
  obstacle : Inport
  Rain : Inport  Port=2
  pass_down : Inport  Port=3
  pass_up : Inport  Port=4
  driver_neutal2 : EnablePort
  passenger : Stateflow chart  TreatAsAtomicUnit=on
  p_up : Outport
  p_down : Outport  Port=2
  wires:
  pass_up/1 -> passenger/4(p_up)  "pass_up"
  pass_down/1 -> passenger/3(p_down)  "pass_down"
  Rain/1 -> passenger/2(Rain)  "Rain"
  passenger/2(Down) -> p_down/1  "p_down"
  passenger/1(Up) -> p_up/1  "p_up"
  obstacle/1 -> passenger/1(Obstacle)  "obstacle"

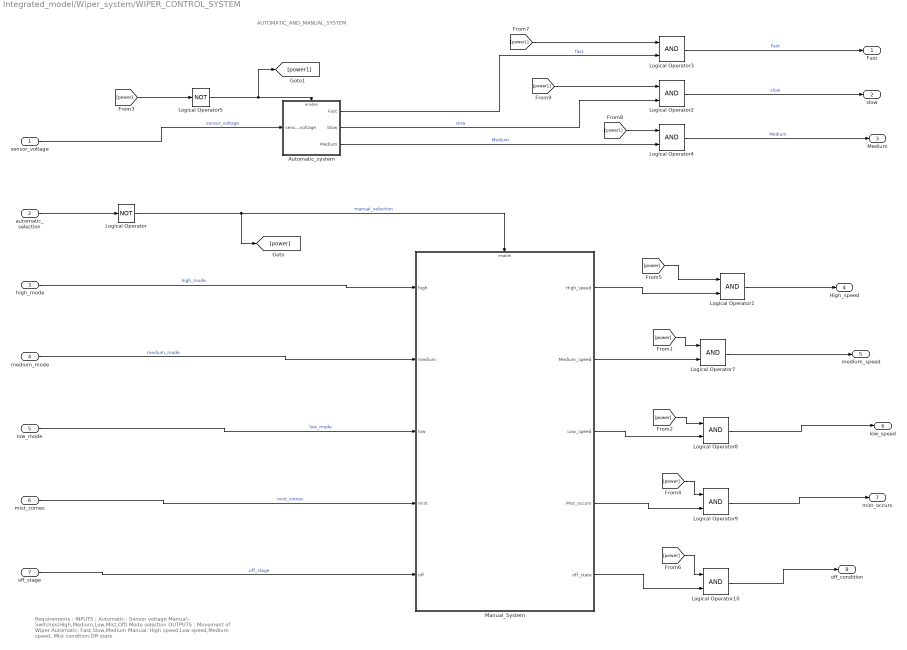
== system Integrated_model/Wiper_system/WIPER_CONTROL_SYSTEM ==
  note: AUTOMATIC_AND_MANUAL_SYSTEM
  note: Requirements :
      |
      | INPUTS :
      | Automatic:-
      | Sensor voltage
      | Manual:-
      | Switches(High,Medium,Low,Mist,Off)
      |
      | Mode selection
      |
      | OUTPUTS :
      | Movement of Wiper
      | Automatic:
      | Fast,Slow,Medium
      | Manual:
      | High speed,Low speed,Medium speed,
      | Mist condition,Off state
  sensor_voltage : Inport
  automatic_selection : Inport  Port=2
  high_mode : Inport  Port=3
  medium_mode : Inport  Port=4
  low_mode : Inport  Port=5
  mist_comes : Inport  Port=6
  off_stage : Inport  Port=7
  Automatic_system : Subsystem
  Logical Operator : Logic  Operator=NOT  AllPortsSameDT=off  OutDataTypeStr=boolean
  Logical Operator{1..4,7..10} (8 alike) : Logic  AllPortsSameDT=off  OutDataTypeStr=boolean
  Logical Operator5 : Logic  Operator=NOT  AllPortsSameDT=off  OutDataTypeStr=boolean
  Manual_System : Subsystem
  Fast : Outport
  slow : Outport  Port=2
  Medium : Outport  Port=3
  High_speed : Outport  Port=4
  medium_speed : Outport  Port=5
  low_speed : Outport  Port=6
  mist_occurs : Outport  Port=7
  off_condition : Outport  Port=8
  wires:
  automatic_selection/1 -> Logical Operator/1
  Manual_System/5(off_state) -> Logical Operator10/2
  [power] -> Logical Operator7/1
  medium_mode/1 -> Manual_System/2(medium)  "medium_mode"
  Logical Operator1/1 -> High_speed/1
  Logical Operator10/1 -> off_condition/1
  Logical Operator9/1 -> mist_occurs/1
  Logical Operator7/1 -> medium_speed/1
  [power] -> Logical Operator8/1
  low_mode/1 -> Manual_System/3(low)  "low_mode"
  mist_comes/1 -> Manual_System/4(mist)  "mist_comes"
  Logical Operator8/1 -> low_speed/1
  Manual_System/3(Low_speed) -> Logical Operator8/2
  Manual_System/1(High_speed) -> Logical Operator1/2
  off_stage/1 -> Manual_System/5(off)  "off_stage"
  [power] -> Logical Operator10/1
  [power] -> Logical Operator1/1
  [power] -> Logical Operator5/1
  Logical Operator/1 -> [power], Manual_System/Enable  "manual_selection"
  Manual_System/4(Mist_occurs) -> Logical Operator9/2
  Manual_System/2(Medium_speed) -> Logical Operator7/2
  [power] -> Logical Operator9/1
  Logical Operator5/1 -> [power1], Automatic_system/Enable
  high_mode/1 -> Manual_System/1(high)  "high_mode"
  sensor_voltage/1 -> Automatic_system/1(sensorvoltage)  "sensor_voltage"
  Automatic_system/1(Fast) -> Logical Operator3/2  "fast"
  Automatic_system/2(Slow) -> Logical Operator2/2  "slow"
  Automatic_system/3(Medium) -> Logical Operator4/2  "Medium"
  [power1] -> Logical Operator3/1
  [power1] -> Logical Operator2/1
  [power1] -> Logical Operator4/1
  Logical Operator3/1 -> Fast/1  "Fast"
  Logical Operator2/1 -> slow/1  "slow"
  Logical Operator4/1 -> Medium/1  "Medium"

== system Integrated_model/Central_lock_System/main_locking_system/fromautomatic ==
  note: AUTOMATIC LOCKING SUBSYSTEM
  note: %REQUIRMENTS::
      | AUTOMATIC LOCKING SYSTEM
      | INPUTS:
      | FROMSPEEDSENSOR
      | FROMGEARSENSOR
      | OUTPUTS:
      | VOLTAGEFROMSENSORS
  speedinput : Inport
  parkinggearinput : Inport  Port=2
  parkinglogic : Switch  Criteria=u2 > Threshold
  speedandparklogic : Sum
  speedlogic : Switch  Criteria=u2 > Threshold
  voltageparkfive : Constant  Value=-5
  voltageparkzero : Constant  Value=0
  voltagespeedfive : Constant  Value=5
  voltagespeedzero : Constant  Value=0
  voltagefromspeedandpark : Outport
  wires:
  speedinput/1 -> speedlogic/2  "speedinput"
  voltagespeedzero/1 -> speedlogic/3
  speedlogic/1 -> speedandparklogic/1  "speedvol"
  parkinglogic/1 -> speedandparklogic/2  "parkvol"
  parkinggearinput/1 -> parkinglogic/2  "parkinggearinput"
  voltageparkzero/1 -> parkinglogic/3
  voltageparkfive/1 -> parkinglogic/1
  voltagespeedfive/1 -> speedlogic/1
  speedandparklogic/1 -> voltagefromspeedandpark/1  "voltagefromspeedandpark"

== system Integrated_model/Central_lock_System/main_locking_system/fromemergency ==
  note: EMERGENCY SUB SYSTEM
  note: %REQUIRMENTS:
      | AIRBAG UNLOCKING SUBSYSTEM
      | INPUTS:
      | AIRBAGSENSOR
      | OUTPUTS:
      | VOLTAGE
  airbaginput : Inport
  airbaglogic : Switch  Criteria=u2 > Threshold
  voltageairbag : Constant  Value=-20
  voltagezero : Constant  Value=0
  collisionvol : Outport
  wires:
  voltagezero/1 -> airbaglogic/3
  airbaglogic/1 -> collisionvol/1  "collisionvol"
  voltageairbag/1 -> airbaglogic/1
  airbaginput/1 -> airbaglogic/2  "airbaginput"

== system Integrated_model/Central_lock_System/main_locking_system/frommanual ==
  note: manual locking system
  note: % REQUIRMENTS::
      | MANUAL LOCKING SYSTEM
      | INPUTS:
      | PUSHBUTTON1
      | PUSHBUTTON2
      | OUTPUTS:
      | VOLTAGEFROMBUTTONS
  pushbutton1 : Inport
  pushbutton2 : Inport  Port=2
  pb1logic : Switch  Criteria=u2 > Threshold
  pb2logic : Switch  Criteria=u2 > Threshold
  pushbuttonvoltage : Sum
  voltagepb1five : Constant  Value=5
  voltagepb1zero : Constant  Value=0
  voltagepb2five : Constant  Value=-5
  voltagepb2zero : Constant  Value=0
  voltagefrombuttons : Outport
  wires:
  pushbutton2/1 -> pb2logic/2  "pushbutton2"
  voltagepb1five/1 -> pb1logic/1
  pushbutton1/1 -> pb1logic/2  "pushbutton1"
  voltagepb1zero/1 -> pb1logic/3
  pb2logic/1 -> pushbuttonvoltage/2  "pb2"
  voltagepb2five/1 -> pb2logic/1
  voltagepb2zero/1 -> pb2logic/3
  pb1logic/1 -> pushbuttonvoltage/1  "pb1"
  pushbuttonvoltage/1 -> voltagefrombuttons/1  "voltagefrombuttons"

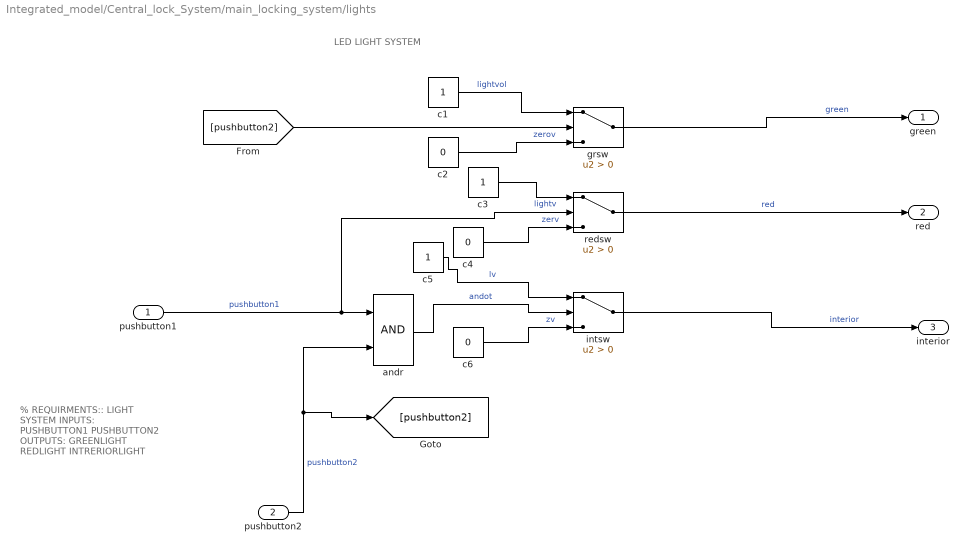
== system Integrated_model/Central_lock_System/main_locking_system/lights ==
  note: LED LIGHT SYSTEM
  note: % REQUIRMENTS::
      | LIGHT SYSTEM
      | INPUTS:
      | PUSHBUTTON1
      | PUSHBUTTON2
      | OUTPUTS:
      | GREENLIGHT
      | REDLIGHT
      | INTRERIORLIGHT
  pushbutton1 : Inport
  pushbutton2 : Inport  Port=2
  andr : Logic  AllPortsSameDT=off  OutDataTypeStr=boolean
  c1 : Constant
  c2 : Constant  Value=0
  c3 : Constant
  c4 : Constant  Value=0
  c5 : Constant
  c6 : Constant  Value=0
  grsw : Switch  Criteria=u2 > Threshold
  intsw : Switch  Criteria=u2 > Threshold
  redsw : Switch  Criteria=u2 > Threshold
  green : Outport
  red : Outport  Port=2
  interior : Outport  Port=3
  wires:
  c6/1 -> intsw/3  "zv"
  c5/1 -> intsw/1  "lv"
  andr/1 -> intsw/2  "andot"
  pushbutton1/1 -> redsw/2, andr/1  "pushbutton1"
  intsw/1 -> interior/1  "interior"
  pushbutton2/1 -> [pushbutton2], andr/2  "pushbutton2"
  grsw/1 -> green/1  "green"
  c1/1 -> grsw/1  "lightvol"
  redsw/1 -> red/1  "red"
  c2/1 -> grsw/3  "zerov"
  c3/1 -> redsw/1  "lightv"
  c4/1 -> redsw/3  "zerv"
  [pushbutton2] -> grsw/2

== system Integrated_model/Central_lock_System/main_locking_system/voltagecombiner ==
  note: VOLTAGECALCULATOR
  note: %REQUIRMENTS:
      | FINALADDER
      | INPUTS:
      | OUTPUTS OF 3 SUBSYSTEMS
      | OUTPUTS:
      | FINALVALUETOMOTOR
  pbvolt : Inport
  parkspeedvol : Inport  Port=2
  airbagvol : Inport  Port=3
  finalviltagecalculation : Sum  Inputs=+++
  to_lock_unlock : Stateflow chart  TreatAsAtomicUnit=on
  status : Outport
  wires:
  parkspeedvol/1 -> finalviltagecalculation/2  "parkspeedvol"
  airbagvol/1 -> finalviltagecalculation/3  "airbagvol"
  pbvolt/1 -> finalviltagecalculation/1  "pbvolt"
  to_lock_unlock/1(status) -> status/1  "status"
  finalviltagecalculation/1 -> to_lock_unlock/1(finalvoltage)  "finalvoltage"

== system Integrated_model/HVAC_System/HVAC_System/Automatic_Manual_system ==
  note: Automatic_Manual_Control_Block
  note: %age Requirements
      |
      | input1: Auto-manual control signal
      | input2: user temp value
      | input3: sensor temp value.
      | input4: Humidity sensor input
      | output1: Final temperature output
      | output2: Dehumidifying value
      | logic: System will give the logical output as per
      | the automation mode
  AutoManualSignal : Inport
  ManualInpts : Inport  Port=2
  Temperature : Inport  Port=3
  HumiditySensor : Inport  Port=4
  Add : Sum
  Automatic_Model : Subsystem
  Manual_Model : Subsystem
  Product : Product
  FinaltempValue : Outport
  DehumidfyingValue : Outport  Port=2
  wires:
  Manual_Model/1(ManualValue) -> Add/1  "ManualValue"
  Manual_Model/2(autocontrol) -> Product/1, Automatic_Model/Enable  "autocontrol"
  AutoManualSignal/1 -> Manual_Model/1(AutoManualSignal)  "AutoManualSignal"
  ManualInpts/1 -> Manual_Model/2(ManualInpts)  "ManualInpts"
  Add/1 -> FinaltempValue/1  "FinaltempValue"
  Temperature/1 -> Automatic_Model/1(Temperature)  "Temperature"
  Automatic_Model/2(DehumidfyingValue) -> DehumidfyingValue/1  "DehumidfyingValue"
  HumiditySensor/1 -> Automatic_Model/2(HumiditySensor)  "HumiditySensor"
  Automatic_Model/1(Tvalue) -> Product/2  "Tvalue"
  Product/1 -> Add/2

== system Integrated_model/HVAC_System/HVAC_System/MotorSpeed_Calcn ==
  note: Motor_Speed_Control_Block
  note: %age Requirements
      | inputs: high low voltage signals
      | outputs: motor speed
      | logic: Value is converted to motor speed
      | using suitable techniques
  FinaltempValue : Inport
  DehumudifyingValue : Inport  Port=2
  Dehumid_motor_Speed : Subsystem
  temp_to_motorSpeed : Subsystem
  HeaterMotorSpeed : Outport
  CoolerMotorSpeed : Outport  Port=2
  DehumidMotorSpeed : Outport  Port=3
  wires:
  Dehumid_motor_Speed/1(Dehumidifyingspeed) -> DehumidMotorSpeed/1  "DehumidMotorSpeed"
  DehumudifyingValue/1 -> Dehumid_motor_Speed/1(DehumidifyingValue)  "DehumudifyingValue"
  temp_to_motorSpeed/1(HeaterMotorSpeed) -> HeaterMotorSpeed/1  "HeaterMotorSpeed"
  temp_to_motorSpeed/2(CoolerMotorSpeed) -> CoolerMotorSpeed/1  "CoolerMotorSpeed"
  FinaltempValue/1 -> temp_to_motorSpeed/1(temp_input)  "FinaltempValue"

== system Integrated_model/HVAC_System/HVAC_System/PWM_Converter ==
  note: Motorspeeed_to_PWM_Converter
  note: %age Requirements
      |
      | input:motorspeed
      | output: pwm
      | logic: motorspeed is converted to PWM
      | by multiplying to corresponding n-bit ADC.
      | ( Note: Considered for a 10 bit ADC )
  HeaterMotorSpeed : Inport
  ADC_block : Constant  Value=2^nBitConverter
  Add : Sum  Inputs=+-
  Constant : Constant
  Constant1 : Constant  Value=0
  Data Type Conversion : DataTypeConversion
  Duty_to_PWM : Product
  DutycycleCalc : Gain  Gain=1/H_Speed
  Switch : Switch  Criteria=u2 ~= 0
  Heater_PWM : Outport
  wires:
  HeaterMotorSpeed/1 -> DutycycleCalc/1  "HeaterMotorSpeed"
  ADC_block/1 -> Duty_to_PWM/2  "nbit"
  DutycycleCalc/1 -> Duty_to_PWM/1  "Dutycycle"
  Duty_to_PWM/1 -> Add/1
  Constant/1 -> Add/2
  Add/1 -> Data Type Conversion/1
  Data Type Conversion/1 -> Switch/1, Switch/2  "MotorPWM"
  Constant1/1 -> Switch/3
  Switch/1 -> Heater_PWM/1  "Heater_PWM"

== system Integrated_model/HVAC_System/HVAC_System/PWM_Converter1 ==
  note: Motorspeeed_to_PWM_Converter
  note: %age Requirements
      |
      | input:motorspeed
      | output: pwm
      | logic: motorspeed is converted to PWM
      | by multiplying to corresponding n-bit ADC.
      | ( Note: Considered for a 10 bit ADC )
  CoolerMotorSpeed : Inport
  ADC_block : Constant  Value=2^nBitConverter
  Add : Sum  Inputs=+-
  Constant : Constant
  Constant1 : Constant  Value=0
  Data Type Conversion : DataTypeConversion
  Duty_to_PWM : Product
  DutycycleCalc : Gain  Gain=1/H_Speed
  Switch : Switch  Criteria=u2 ~= 0
  Cooler_PWM : Outport
  wires:
  CoolerMotorSpeed/1 -> DutycycleCalc/1  "CoolerMotorSpeed"
  ADC_block/1 -> Duty_to_PWM/2  "nbit"
  DutycycleCalc/1 -> Duty_to_PWM/1  "Dutycycle"
  Duty_to_PWM/1 -> Add/1
  Constant/1 -> Add/2
  Add/1 -> Data Type Conversion/1
  Data Type Conversion/1 -> Switch/1, Switch/2  "MotorPWM"
  Constant1/1 -> Switch/3
  Switch/1 -> Cooler_PWM/1  "Cooler_PWM"

== system Integrated_model/HVAC_System/HVAC_System/PWM_Converter2 ==
  note: Motorspeeed_to_PWM_Converter
  note: %age Requirements
      |
      | input:motorspeed
      | output: pwm
      | logic: motorspeed is converted to PWM
      | by multiplying to corresponding n-bit ADC.
      | ( Note: Considered for a 10 bit ADC )
  DehumidMotorSpeed : Inport
  ADC_block : Constant  Value=2^nBitConverter
  Add : Sum  Inputs=+-
  Constant : Constant
  Constant1 : Constant  Value=0
  Data Type Conversion : DataTypeConversion
  Duty_to_PWM : Product
  DutycycleCalc : Gain  Gain=1/H_Speed
  Switch : Switch  Criteria=u2 ~= 0
  Dehumid_PWM : Outport
  wires:
  DehumidMotorSpeed/1 -> DutycycleCalc/1  "DehumidMotorSpeed"
  ADC_block/1 -> Duty_to_PWM/2  "nbit"
  DutycycleCalc/1 -> Duty_to_PWM/1  "Dutycycle"
  Duty_to_PWM/1 -> Add/1
  Constant/1 -> Add/2
  Add/1 -> Data Type Conversion/1
  Data Type Conversion/1 -> Switch/1, Switch/2  "MotorPWM"
  Constant1/1 -> Switch/3
  Switch/1 -> Dehumid_PWM/1  "Dehumid_PWM"

== system Integrated_model/HVAC_System/HVAC_System/SensorVoltage_to_Temperature ==
  note: %age Requirements
      |
      | input:voltage
      | output:Temperature
      | logic: Sensor Voltage is converted to temperture
      | using proper equation
      | (Temperature Sensor assumed: TMP36 )
  note: SensorVoltage_to_Temperature_Conversion
  TemperatureSensorinputs : Inport
  CaliberatedValue : Gain  Gain=1/10
  Constant4 : Constant  Value=500
  Negation : Sum  Inputs=+-
  Volt_to_mV : Gain  Gain=1000
  Temperature : Outport
  wires:
  Volt_to_mV/1 -> Negation/1  "valuein_mV"
  Constant4/1 -> Negation/2
  CaliberatedValue/1 -> Temperature/1  "Temperature"
  TemperatureSensorinputs/1 -> Volt_to_mV/1  "TemperatureSensorinputs"
  Negation/1 -> CaliberatedValue/1  "negatedvolatge"

== system Integrated_model/Lighting_System/Automode/Conversion_system ==
  In_Lux : Inport
  Constant : Constant
  Constant1 : Constant  Value=0
  Saturation : Saturate  UpperLimit=20  LowerLimit=10
      settings: AttributesFormatString=|
      | %<UpperLimit>
      | %<LowerLimit>
  Saturation1 : Saturate  UpperLimit=200  LowerLimit=150
      settings: AttributesFormatString=|
      | %<UpperLimit>
      | %<LowerLimit>
  Switch : Switch  Criteria=u2 > Threshold  Threshold=15
      settings: AttributesFormatString=%<Threshold>
  In_Street_Light : Outport
  In_Reflection_opposite_vehicle : Outport  Port=2
  wires:
  Constant1/1 -> Switch/3
  Switch/1 -> In_Street_Light/1  "In_Street_Light"
  Saturation/1 -> Switch/2
  Constant/1 -> Switch/1
  Saturation1/1 -> In_Reflection_opposite_vehicle/1  "In_Reflection_opposite_vehicle"
  In_Lux/1 -> Saturation1/1, Saturation/1  "In_Lux"

== system Integrated_model/Lighting_System/Automode/For_BackLight ==
  note: %REQUIREMENTS:
      | INPUT:
      | -> Pressure
      | OUTPUT:
      | ->BackLight Intensity
  In_Pressure : Inport
  Constant : Constant  Value=0
  Constant1 : Constant
  Switch : Switch  Criteria=u2 > Threshold  Threshold=0.6
      settings: AttributesFormatString=%<Threshold>
  v : Lookup_n-D  NumberOfTableDimensions=1  BreakpointsForDimension1=[0 300]  Table=[0 5]  InternalRulePriority=Speed  RndMeth=Simplest  InputSameDT=on
      settings: AttributesFormatString=%<RndMeth>Floor
  Out_Intensity : Outport
  wires:
  v/1 -> Switch/2  "v"
  In_Pressure/1 -> v/1  "In_Pressure"
  Switch/1 -> Out_Intensity/1  "Out_Intensity"
  Constant1/1 -> Switch/1
  Constant/1 -> Switch/3

== system Integrated_model/Lighting_System/Automode/HeadLight_and_DayLight ==
  In_Distance_sensor : Inport
  In_Street_Light : Inport  Port=2
  In_Reflection_opposite_vehicle : Inport  Port=3
  In_Light_Intensity : Inport  Port=4
  FOr_comparing_with_daylight : Subsystem
  For_COmparision_with_Daylight : Subsystem
  For_HeadLight : Subsystem
  Out_High_Beam : Outport
  Out_Low_Beam : Outport  Port=2
  wires:
  In_Light_Intensity/1 -> For_COmparision_with_Daylight/1(In_Intensity), FOr_comparing_with_daylight/2(In_Light_Intensity)  "In_Light_Intensity"
  In_Street_Light/1 -> For_HeadLight/2(InStreet_Light)  "In_Street_Light"
  In_Reflection_opposite_vehicle/1 -> For_HeadLight/3(InReflection_opposite_vehicle)  "In_Reflection_opposite_vehicle"
  In_Distance_sensor/1 -> For_HeadLight/1(In_Distance_sensor)  "In_Distance_sensor"
  For_HeadLight/1(Out_High_beam_1) -> FOr_comparing_with_daylight/1(Out_High_beam_1)  "Out_High_beam_1"
  FOr_comparing_with_daylight/1(Out_High_Beam) -> Out_High_Beam/1  "Out_High_Beam"
  For_HeadLight/2(Out_Low_Beam_2) -> For_COmparision_with_Daylight/2(Out_Low_Beam_2)  "Out_Low_Beam_2"
  For_COmparision_with_Daylight/1(Out_Low_Beam) -> Out_Low_Beam/1  "Out_Low_Beam"

== system Integrated_model/Lighting_System/Automode/Light_Indicator_ ==
  note: %REQUIREMENTS:
      | Input:
      | ->Luminous_intensity
      | Output:
      | ->Maintainable_Intensity
  In_Lux : Inport
  Day_light_intense : Stateflow chart  TreatAsAtomicUnit=on
  f : Lookup_n-D  NumberOfTableDimensions=1  BreakpointsForDimension1=[0 800]  Table=[0 3]  InternalRulePriority=Speed  RndMeth=Simplest  InputSameDT=on
      settings: AttributesFormatString=%<RndMeth>Floor
  In_Light_Intensity : Outport
  wires:
  Day_light_intense/1(In_Light_Intensity) -> In_Light_Intensity/1  "In_Light_Intensity"
  In_Lux/1 -> f/1  "In_Lux"
  f/1 -> Day_light_intense/1(f)  "f"

== system Integrated_model/Wiper_system/WIPER_CONTROL_SYSTEM/Automatic_system ==
  note: AUTOMATIC_WIPER_SYSTEM
  note: Requirements :
      |
      | INPUTS :
      | Sensor voltage
      |
      | OUTPUTS :
      | Movement of Wiper
      | Automatic:
      | Fast,Slow,Medium
      |
      | LOGIC :
      | State flow chart
  sensorvoltage : Inport
  Enable : EnablePort
  conditions : Stateflow chart  TreatAsAtomicUnit=on
  voltage_to_intensity : Lookup_n-D  NumberOfTableDimensions=1  BreakpointsForDimension1=[0 10]  Table=[40 130]  InternalRulePriority=Speed  RndMeth=Simplest  InputSameDT=on
      settings: AttributesFormatString=%<RndMeth>
  Fast : Outport
  Slow : Outport  Port=2
  Medium : Outport  Port=3
  wires:
  voltage_to_intensity/1 -> conditions/1(automatic)
  conditions/1(High) -> Fast/1
  conditions/2(Low) -> Slow/1
  conditions/3(Medium) -> Medium/1
  sensorvoltage/1 -> voltage_to_intensity/1  "sensorvoltage"

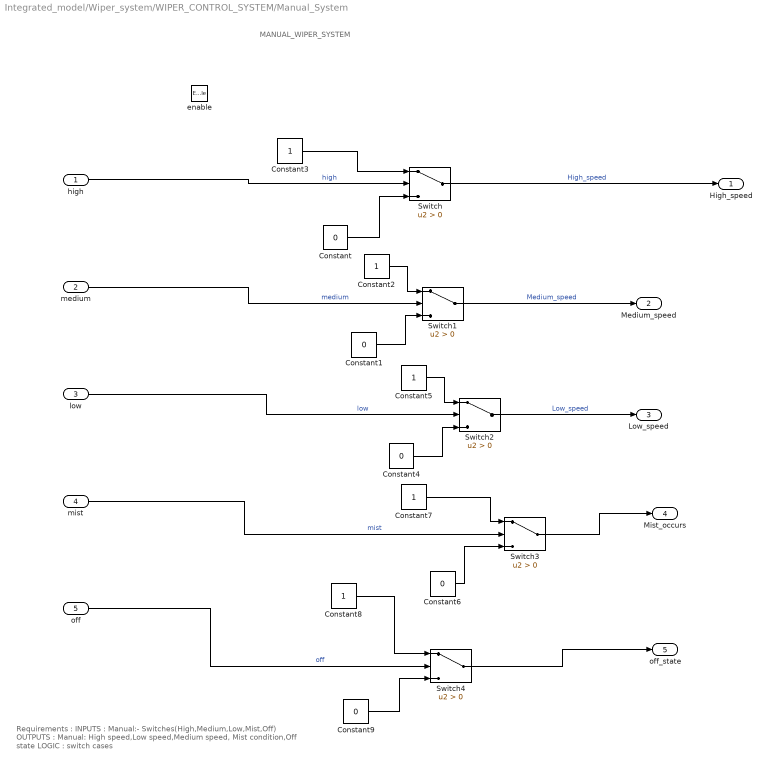
== system Integrated_model/Wiper_system/WIPER_CONTROL_SYSTEM/Manual_System ==
  note: MANUAL_WIPER_SYSTEM
  note: Requirements :
      |
      | INPUTS :
      | Manual:-
      | Switches(High,Medium,Low,Mist,Off)
      |
      | OUTPUTS :
      | Manual:
      | High speed,Low speed,Medium speed,
      | Mist condition,Off state
      |
      | LOGIC :
      | switch cases
  high : Inport
  medium : Inport  Port=2
  low : Inport  Port=3
  mist : Inport  Port=4
  off : Inport  Port=5
  enable : EnablePort
  Constant{,1,4,6,9} (5 alike) : Constant  Value=0
  Constant{2..3,5,7..8} (5 alike) : Constant
  Switch{,1..4} (5 alike) : Switch  Criteria=u2 > Threshold
  High_speed : Outport
  Medium_speed : Outport  Port=2
  Low_speed : Outport  Port=3
  Mist_occurs : Outport  Port=4
  off_state : Outport  Port=5
  wires:
  mist/1 -> Switch3/2  "mist"
  Switch1/1 -> Medium_speed/1  "Medium_speed"
  Constant7/1 -> Switch3/1
  Constant6/1 -> Switch3/3
  Constant/1 -> Switch/3
  Constant8/1 -> Switch4/1
  Constant3/1 -> Switch/1
  Constant5/1 -> Switch2/1
  Constant2/1 -> Switch1/1
  medium/1 -> Switch1/2  "medium"
  Constant4/1 -> Switch2/3
  Constant9/1 -> Switch4/3
  Constant1/1 -> Switch1/3
  Switch/1 -> High_speed/1  "High_speed"
  Switch2/1 -> Low_speed/1  "Low_speed"
  low/1 -> Switch2/2  "low"
  off/1 -> Switch4/2  "off"
  Switch4/1 -> off_state/1
  Switch3/1 -> Mist_occurs/1
  high/1 -> Switch/2  "high"

== system Integrated_model/HVAC_System/HVAC_System/Automatic_Manual_system/Automatic_Model ==
  note: Temperature_to_Motor_Input_Value
  note: %age requirements
      |
      | input 1: Temperature
      | input 2: Humidity
      | output1: System temperature values
      | output2: dehumidifier values
      | logic:
      | HVAC temp is decided from the temperature
      | sensors readings if it is in automatic mode
  Temperature : Inport
  HumiditySensor : Inport  Port=2
  autocontrol : EnablePort
  Temp_sensor_to_Tvalue : Stateflow chart  TreatAsAtomicUnit=on
  int_block : DataTypeConversion  OutDataTypeStr=int8
  int_block1 : DataTypeConversion  OutDataTypeStr=int8
  Tvalue : Outport
  DehumidfyingValue : Outport  Port=2
  wires:
  Temp_sensor_to_Tvalue/1(Tvalue) -> Tvalue/1  "Tvalue"
  Temp_sensor_to_Tvalue/2(DeH) -> DehumidfyingValue/1  "DehumidfyingValue"
  Temperature/1 -> int_block/1  "Temperature"
  HumiditySensor/1 -> int_block1/1  "HumiditySensor"
  int_block/1 -> Temp_sensor_to_Tvalue/1(T)  "T"
  int_block1/1 -> Temp_sensor_to_Tvalue/2(DH)  "DH"

== system Integrated_model/HVAC_System/HVAC_System/Automatic_Manual_system/Manual_Model ==
  note: Manual_Control_Block
  note: %age Requirements
      |
      | input1:control signal
      | input2: manual temperature
      | output: final manual value.
      | logic: if manual control is on,then it will take the
      | manual input by user
  AutoManualSignal : Inport
  ManualInpts : Inport  Port=2
  Data Type Conversion : DataTypeConversion  OutDataTypeStr=boolean
  ManualSwitch : Subsystem
  ManualValue : Outport
  autocontrol : Outport  Port=2
  wires:
  Data Type Conversion/1 -> autocontrol/1, ManualSwitch/1(autocontrol)  "autocontrol"
  AutoManualSignal/1 -> Data Type Conversion/1  "AutoManualSignal"
  ManualInpts/1 -> ManualSwitch/2(ManualInpts)  "ManualInpts"
  ManualSwitch/1(ManualValue) -> ManualValue/1  "ManualValue"

== system Integrated_model/HVAC_System/HVAC_System/MotorSpeed_Calcn/Dehumid_motor_Speed ==
  note: Dehumidifier_Speed
  note: %age Requirements
      |
      | input: Dehumidfyingvalue
      | output: Motor speed
      | logic: Motor speed is given as
      | per the dehumidfying value
  DehumidifyingValue : Inport
  Data Type Conversion : DataTypeConversion  OutDataTypeStr=boolean
  HighestMotorValue : Constant  Value=H_limit
  LowestMotorValue : Constant  Value=L_limit
  Switch : Switch  Criteria=u2 ~= 0
  Dehumidifyingspeed : Outport
  wires:
  HighestMotorValue/1 -> Switch/1  "HighestMotorspeed"
  LowestMotorValue/1 -> Switch/3  "lowerMotorSpeed"
  DehumidifyingValue/1 -> Data Type Conversion/1  "DehumidifyingValue"
  Switch/1 -> Dehumidifyingspeed/1  "Dehumidifyingspeed"
  Data Type Conversion/1 -> Switch/2  "DehumidifyingValue1"
